simulink model "Controle_UDP_0809_simulador"  (R2014a)
settings: Solver=ode45  StartTime=0.0  StopTime=360  RelTol=1e-3
values from neighbouring files (symbols this model uses):
  Arwx = [-B1/J1 Kt/J1 ... (first row only)    [data_ACS_HIL.m]
  Arwy = [-B2/J2 Kt/J2 ... (first row only)    [data_ACS_HIL.m]
  Arwz = [-B3/J3 Kt/J3 ... (first row only)    [data_ACS_HIL.m]
  Brwx = [0 ... (first row only)    [data_ACS_HIL.m]
  Brwy = [0 ... (first row only)    [data_ACS_HIL.m]
  Brwz = [0 ... (first row only)    [data_ACS_HIL.m]
  Crwx = [1 0 ... (first row only)    [data_ACS_HIL.m]
  Crwy = [1 0 ... (first row only)    [data_ACS_HIL.m]
  Crwz = [1 0 ... (first row only)    [data_ACS_HIL.m]
  Drwx = zeros(3,1)    [data_ACS_HIL.m]
  Drwy = zeros(3,1)    [data_ACS_HIL.m]
  Drwz = zeros(3,1)    [data_ACS_HIL.m]
  I1 = 0.000624567    [data_ACS_HIL.m]
  I2 = 0.000624567    [data_ACS_HIL.m]
  I3 = 0.000624567    [data_ACS_HIL.m]
  in1 = [ 10 10 25 30 0 ] * pi / 180    [data_ACS_HIL.m]
  in2 = [ 0 10 10 30 0 ] * pi / 180    [data_ACS_HIL.m]
  in3 = [ 45 -30 30 30 0 ] * pi / 180    [data_ACS_HIL.m]
  Ixx = I( 1, 1 )    [data_ACS_HIL.m]
  Iyy = I( 2, 2 )    [data_ACS_HIL.m]
  Izz = I( 3, 3 )    [data_ACS_HIL.m]
  J1 = I1 + 3e-06    (= 0.000627567)    [data_ACS_HIL.m]
  J2 = I2 + 3e-06    (= 0.000627567)    [data_ACS_HIL.m]
  J3 = I3 + 3e-06    (= 0.000627567)    [data_ACS_HIL.m]
  Ki_x = 1    [data_ACS_HIL.m]
  Ki_y = Ki_x    (= 1)    [data_ACS_HIL.m]
  Ki_z = Ki_x    (= 1)    [data_ACS_HIL.m]
  Kp_x = 0.2    [data_ACS_HIL.m]
  Kp_y = Kp_x    (= 0.2)    [data_ACS_HIL.m]
  Kp_z = Kp_x    (= 0.2)    [data_ACS_HIL.m]
  Kpx = vp * (wn^2) * Ixx    [data_ACS_HIL.m]
  Kpy = vp * (wn^2) * Iyy    [data_ACS_HIL.m]
  Kpz = vp * (wn^2) * Izz    [data_ACS_HIL.m]
  Krx = vr * 2 * Ixx * wn * qsi    [data_ACS_HIL.m]
  Kry = vr * 2 * Iyy * wn * qsi    [data_ACS_HIL.m]
  Krz = vr * 2 * Izz * wn * qsi    [data_ACS_HIL.m]
  mW0 = 0000 / ( 60 / ( 2*pi ) )    (= 0)    [data_ACS_HIL.m]
  Wx0 = [mW0 0]    [data_ACS_HIL.m]
  Wy0 = [mW0 0]    [data_ACS_HIL.m]
  Wz0 = [mW0 0]    [data_ACS_HIL.m]
libraries: aerolibconvert2 x6, simulink x6, etargetslib x4, instrumentlib x4, aerolibutil x4, xpcutilitieslib x2, slrtlib x2, rtwinlib x1, aerolibtransform2 x1, vrlib x1
(part 2 of 2)

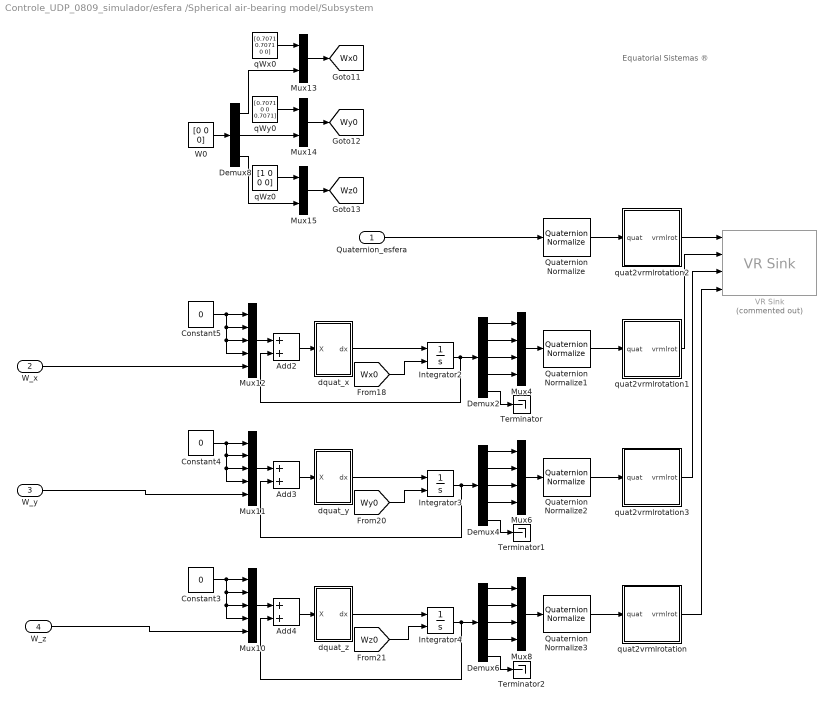
== system Controle_UDP_0809_simulador/esfera /Spherical air-bearing model/Subsystem ==
  note: Equatorial Sistemas ®
  Quaternion_esfera : Inport
  W_x : Inport  Port=2
  W_y : Inport  Port=3
  W_z : Inport  Port=4
  Add2 : Sum
  Add3 : Sum
  Add4 : Sum
  Constant3 : Constant  Value=0
  Constant4 : Constant  Value=0
  Constant5 : Constant  Value=0
  Demux2 : Demux  Outputs=5
  Demux4 : Demux  Outputs=5
  Demux6 : Demux  Outputs=5
  Demux8 : Demux  Outputs=3
  Integrator2 : Integrator  InitialConditionSource=external  InitialCondition=Wx0
  Integrator3 : Integrator  InitialConditionSource=external  InitialCondition=Wy0
  Integrator4 : Integrator  InitialConditionSource=external  InitialCondition=Wz0
  Mux10 : Mux  Inputs=5
  Mux11 : Mux  Inputs=5
  Mux12 : Mux  Inputs=5
  Mux13 : Mux  Inputs=2
  Mux14 : Mux  Inputs=2
  Mux15 : Mux  Inputs=2
  Mux4 : Mux
  Mux6 : Mux
  Mux8 : Mux
  Quaternion Normalize{,1..3} (4 alike) : aerolibutil/Quaternion Normalize
  Terminator : Terminator
  Terminator1 : Terminator
  Terminator2 : Terminator
  VR Sink : vrlib/VR Sink  Commented=on  InstantiateOnLoad=on  SampleTime=0.1  ViewEnable=on  RemoteChange=off  RemoteView=off  FieldsWritten=Corpo.rotation.4.1.1.double#Roda_x.rotation.4.1.1.double#Roda_y.rotation.4.1.1.double#Roda_z.rotation.4.1.1.double  WorldFileName=wrlfiles\esfera_v2.wrl  WorldDescription=VRML MATLAB Membrane  AutoView=on  VideoDimensions=[]  AllowVariableSize=off
  W0 : Constant  Value=[0 0 0]
  dquat_x : Subsystem
  dquat_y : Subsystem
  dquat_z : Subsystem
  qWx0 : Constant  Value=[0.7071 0.7071 0 0]
  qWy0 : Constant  Value=[0.7071 0 0 0.7071]
  qWz0 : Constant  Value=[1 0 0 0]
  quat2vrmlrotation : Subsystem
  quat2vrmlrotation1 : Subsystem
  quat2vrmlrotation2 : Subsystem
  quat2vrmlrotation3 : Subsystem
  tag scope: Wx0=global, Wy0=global, Wz0=global
  wires:
  Integrator2/1 -> Demux2/1, Add2/2
  Mux4/1 -> Quaternion Normalize1/1
  Add2/1 -> dquat_x/1(X)
  Demux2/1 -> Mux4/1
  Demux2/2 -> Mux4/2
  Demux2/3 -> Mux4/3
  Demux2/4 -> Mux4/4
  Integrator3/1 -> Demux4/1, Add3/2
  Mux6/1 -> Quaternion Normalize2/1
  Demux4/1 -> Mux6/1
  Demux4/2 -> Mux6/2
  Demux4/3 -> Mux6/3
  Demux4/4 -> Mux6/4
  Integrator4/1 -> Add4/2, Demux6/1
  Mux8/1 -> Quaternion Normalize3/1
  Quaternion Normalize3/1 -> quat2vrmlrotation/1(quat)
  Demux6/1 -> Mux8/1
  Demux6/2 -> Mux8/2
  Demux6/3 -> Mux8/3
  Demux6/4 -> Mux8/4
  Mux10/1 -> Add4/1
  Mux11/1 -> Add3/1
  Constant5/1 -> Mux12/1, Mux12/2, Mux12/3, Mux12/4
  Mux12/1 -> Add2/1
  Constant4/1 -> Mux11/1, Mux11/2, Mux11/3, Mux11/4
  Constant3/1 -> Mux10/1, Mux10/2, Mux10/3, Mux10/4
  [Wx0] -> Integrator2/2
  [Wy0] -> Integrator3/2
  [Wz0] -> Integrator4/2
  W0/1 -> Demux8/1
  qWx0/1 -> Mux13/1
  Demux8/1 -> Mux13/2
  Mux13/1 -> [Wx0]
  qWy0/1 -> Mux14/1
  Demux8/2 -> Mux14/2
  Mux14/1 -> [Wy0]
  qWz0/1 -> Mux15/1
  Demux8/3 -> Mux15/2
  Mux15/1 -> [Wz0]
  dquat_x/1(dx) -> Integrator2/1
  Add3/1 -> dquat_y/1(X)
  dquat_y/1(dx) -> Integrator3/1
  Add4/1 -> dquat_z/1(X)
  dquat_z/1(dx) -> Integrator4/1
  Demux2/5 -> Terminator/1
  Demux4/5 -> Terminator1/1
  Demux6/5 -> Terminator2/1
  Quaternion Normalize/1 -> quat2vrmlrotation2/1(quat)
  Quaternion Normalize1/1 -> quat2vrmlrotation1/1(quat)
  Quaternion Normalize2/1 -> quat2vrmlrotation3/1(quat)
  quat2vrmlrotation2/1(vrmlrot) -> VR Sink/1
  quat2vrmlrotation1/1(vrmlrot) -> VR Sink/2
  quat2vrmlrotation3/1(vrmlrot) -> VR Sink/3
  quat2vrmlrotation/1(vrmlrot) -> VR Sink/4
  W_y/1 -> Mux11/5
  W_z/1 -> Mux10/5
  W_x/1 -> Mux12/5
  Quaternion_esfera/1 -> Quaternion Normalize/1

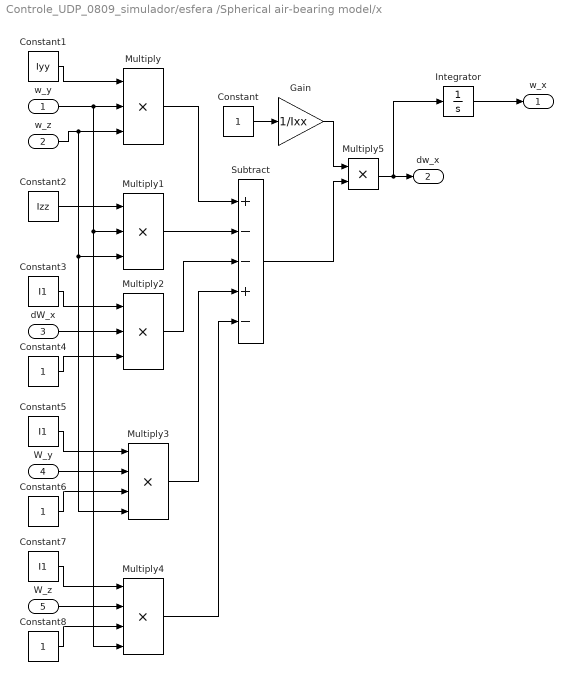
== system Controle_UDP_0809_simulador/esfera /Spherical air-bearing model/x ==
  w_y : Inport
  w_z : Inport  Port=2
  dW_x : Inport  Port=3
  W_y : Inport  Port=4
  W_z : Inport  Port=5
  Constant{,4,6,8} (4 alike) : Constant
  Constant1 : Constant  Value=Iyy
  Constant2 : Constant  Value=Izz
  Constant3 : Constant  Value=I1
  Constant5 : Constant  Value=I1
  Constant7 : Constant  Value=I1
  Gain : Gain  Gain=1/Ixx
  Integrator : Integrator
  Multiply : Product  Inputs=***
  Multiply1 : Product  Inputs=***
  Multiply2 : Product  Inputs=***
  Multiply3 : Product  Inputs=****
  Multiply4 : Product  Inputs=****
  Multiply5 : Product  Inputs=**
  Subtract : Sum  Inputs=+--+-
  w_x : Outport
  dw_x : Outport  Port=2
  wires:
  Constant/1 -> Gain/1
  Gain/1 -> Multiply5/1
  Constant1/1 -> Multiply/1
  Multiply/1 -> Subtract/1
  Constant2/1 -> Multiply1/1
  Multiply1/1 -> Subtract/2
  Constant3/1 -> Multiply2/1
  Constant4/1 -> Multiply2/3
  Multiply2/1 -> Subtract/3
  Constant5/1 -> Multiply3/1
  Constant6/1 -> Multiply3/3
  Constant7/1 -> Multiply4/1
  Constant8/1 -> Multiply4/3
  Multiply3/1 -> Subtract/4
  Multiply4/1 -> Subtract/5
  Subtract/1 -> Multiply5/2
  w_y/1 -> Multiply/2, Multiply1/2, Multiply4/4
  w_z/1 -> Multiply/3, Multiply1/3, Multiply3/4
  dW_x/1 -> Multiply2/2
  W_y/1 -> Multiply3/2
  W_z/1 -> Multiply4/2
  Multiply5/1 -> Integrator/1, dw_x/1
  Integrator/1 -> w_x/1

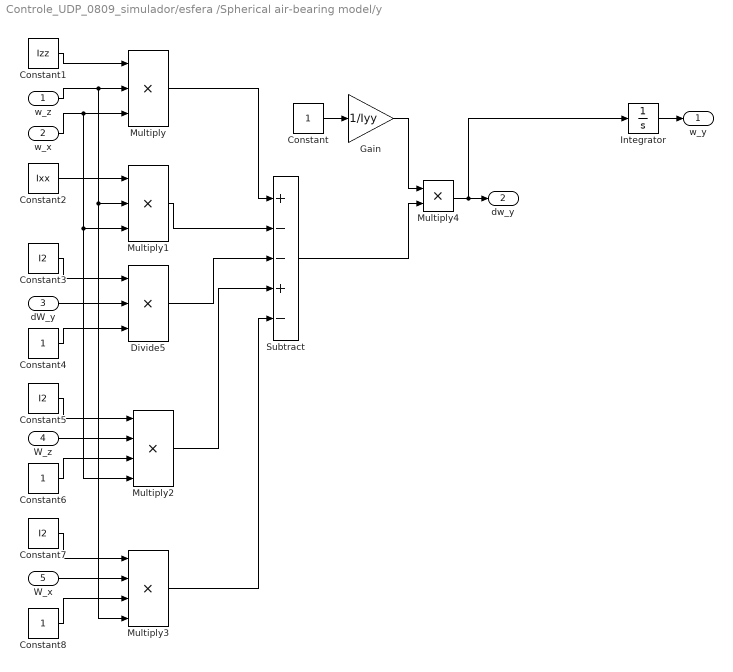
== system Controle_UDP_0809_simulador/esfera /Spherical air-bearing model/y ==
  w_z : Inport
  w_x : Inport  Port=2
  dW_y : Inport  Port=3
  W_z : Inport  Port=4
  W_x : Inport  Port=5
  Constant{,4,6,8} (4 alike) : Constant
  Constant1 : Constant  Value=Izz
  Constant2 : Constant  Value=Ixx
  Constant3 : Constant  Value=I2
  Constant5 : Constant  Value=I2
  Constant7 : Constant  Value=I2
  Divide5 : Product  Inputs=***
  Gain : Gain  Gain=1/Iyy
  Integrator : Integrator
  Multiply : Product  Inputs=***
  Multiply1 : Product  Inputs=***
  Multiply2 : Product  Inputs=****
  Multiply3 : Product  Inputs=****
  Multiply4 : Product  Inputs=**
  Subtract : Sum  Inputs=+--+-
  w_y : Outport
  dw_y : Outport  Port=2
  wires:
  W_x/1 -> Multiply3/2
  W_z/1 -> Multiply2/2
  dW_y/1 -> Divide5/2
  w_x/1 -> Multiply2/4, Multiply1/3, Multiply/3
  w_z/1 -> Multiply3/4, Multiply1/2, Multiply/2
  Subtract/1 -> Multiply4/2
  Multiply3/1 -> Subtract/5
  Multiply2/1 -> Subtract/4
  Constant8/1 -> Multiply3/3
  Constant7/1 -> Multiply3/1
  Constant6/1 -> Multiply2/3
  Constant5/1 -> Multiply2/1
  Divide5/1 -> Subtract/3
  Constant4/1 -> Divide5/3
  Constant3/1 -> Divide5/1
  Multiply1/1 -> Subtract/2
  Constant2/1 -> Multiply1/1
  Multiply/1 -> Subtract/1
  Constant1/1 -> Multiply/1
  Integrator/1 -> w_y/1
  Gain/1 -> Multiply4/1
  Constant/1 -> Gain/1
  Multiply4/1 -> Integrator/1, dw_y/1

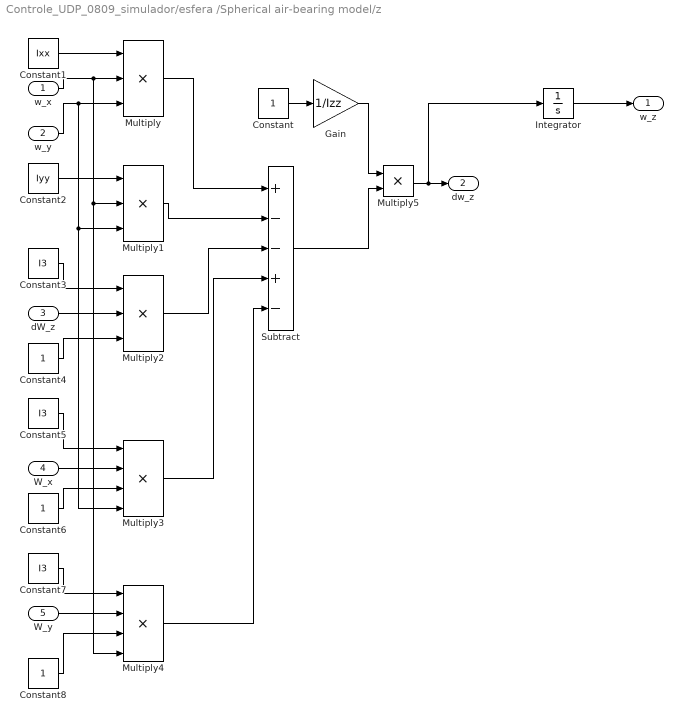
== system Controle_UDP_0809_simulador/esfera /Spherical air-bearing model/z ==
  w_x : Inport
  w_y : Inport  Port=2
  dW_z : Inport  Port=3
  W_x : Inport  Port=4
  W_y : Inport  Port=5
  Constant{,4,6,8} (4 alike) : Constant
  Constant1 : Constant  Value=Ixx
  Constant2 : Constant  Value=Iyy
  Constant3 : Constant  Value=I3
  Constant5 : Constant  Value=I3
  Constant7 : Constant  Value=I3
  Gain : Gain  Gain=1/Izz
  Integrator : Integrator
  Multiply : Product  Inputs=***
  Multiply1 : Product  Inputs=***
  Multiply2 : Product  Inputs=***
  Multiply3 : Product  Inputs=****
  Multiply4 : Product  Inputs=****
  Multiply5 : Product  Inputs=**
  Subtract : Sum  Inputs=+--+-
  w_z : Outport
  dw_z : Outport  Port=2
  wires:
  Constant/1 -> Gain/1
  Gain/1 -> Multiply5/1
  Integrator/1 -> w_z/1
  Constant1/1 -> Multiply/1
  Multiply/1 -> Subtract/1
  Constant2/1 -> Multiply1/1
  Multiply1/1 -> Subtract/2
  Constant3/1 -> Multiply2/1
  Constant4/1 -> Multiply2/3
  Multiply2/1 -> Subtract/3
  Constant5/1 -> Multiply3/1
  Constant6/1 -> Multiply3/3
  Constant7/1 -> Multiply4/1
  Constant8/1 -> Multiply4/3
  Multiply3/1 -> Subtract/4
  Multiply4/1 -> Subtract/5
  Subtract/1 -> Multiply5/2
  w_x/1 -> Multiply/2, Multiply1/2, Multiply4/4
  w_y/1 -> Multiply/3, Multiply1/3, Multiply3/4
  dW_z/1 -> Multiply2/2
  W_x/1 -> Multiply3/2
  W_y/1 -> Multiply4/2
  Multiply5/1 -> Integrator/1, dw_z/1

== system Controle_UDP_0809_simulador/controle /Logica de controle/Logica de Controle/subtrator de angulos ==
  + : Inport
  - : Inport  Port=2
  Constant2 : Constant  Value=2*pi
  Gain : Gain  Gain=-1
  Sum : Sum  Inputs=|+-
  Sum1 : Sum  Inputs=|+-
  Sum2 : Sum  Inputs=|++
  Switch : Switch  Criteria=u2 > Threshold  Threshold=180*pi/180
  Switch1 : Switch  Criteria=u2 > Threshold  Threshold=180*pi/180
  Out1 : Outport
  wires:
  Sum2/1 -> Switch1/1
  Gain/1 -> Switch1/2
  Sum/1 -> Switch/3, Switch/2, Sum1/1
  Sum1/1 -> Switch/1
  Switch/1 -> Switch1/3, Gain/1, Sum2/1
  Constant2/1 -> Sum1/2, Sum2/2
  Switch1/1 -> Out1/1
  -/1 -> Sum/2
  +/1 -> Sum/1

== system Controle_UDP_0809_simulador/esfera /Spherical air-bearing model/Subsystem/dquat_x ==
  X : Inport
  Constant : Constant  Value=0
  Demux : Demux  Outputs=5
  Gain : Gain  Gain=1/2
  Gain1 : Gain  Gain=-1
  Gain2 : Gain  Gain=-1
  Mux : Mux  Inputs=5
  Product{,1..3} (4 alike) : Product
  dx : Outport
  wires:
  X/1 -> Gain/1
  Gain1/1 -> Product/1
  Product1/1 -> Mux/2
  Product2/1 -> Mux/3
  Product3/1 -> Mux/4
  Gain/1 -> Demux/1
  Product/1 -> Mux/1
  Demux/5 -> Product/2, Product1/2, Product2/2, Product3/2
  Mux/1 -> dx/1
  Constant/1 -> Mux/5
  Demux/3 -> Gain1/1
  Gain2/1 -> Product1/1
  Demux/4 -> Gain2/1
  Demux/1 -> Product2/1
  Demux/2 -> Product3/1

== system Controle_UDP_0809_simulador/esfera /Spherical air-bearing model/Subsystem/dquat_y ==
  X : Inport
  Constant : Constant  Value=0
  Demux : Demux  Outputs=5
  Gain : Gain  Gain=1/2
  Gain1 : Gain  Gain=-1
  Gain2 : Gain  Gain=-1
  Mux : Mux  Inputs=5
  Product{,1..3} (4 alike) : Product
  dx : Outport
  wires:
  X/1 -> Gain/1
  Gain1/1 -> Product/1
  Product1/1 -> Mux/2
  Product2/1 -> Mux/3
  Product3/1 -> Mux/4
  Gain/1 -> Demux/1
  Product/1 -> Mux/1
  Demux/5 -> Product/2, Product1/2, Product2/2, Product3/2
  Mux/1 -> dx/1
  Constant/1 -> Mux/5
  Demux/3 -> Gain1/1
  Gain2/1 -> Product1/1
  Demux/4 -> Gain2/1
  Demux/1 -> Product2/1
  Demux/2 -> Product3/1

== system Controle_UDP_0809_simulador/esfera /Spherical air-bearing model/Subsystem/dquat_z ==
  X : Inport
  Constant : Constant  Value=0
  Demux : Demux  Outputs=5
  Gain : Gain  Gain=1/2
  Gain1 : Gain  Gain=-1
  Gain2 : Gain  Gain=-1
  Mux : Mux  Inputs=5
  Product{,1..3} (4 alike) : Product
  dx : Outport
  wires:
  X/1 -> Gain/1
  Gain1/1 -> Product/1
  Product1/1 -> Mux/2
  Product2/1 -> Mux/3
  Product3/1 -> Mux/4
  Demux/1 -> Product2/1
  Demux/3 -> Gain1/1
  Demux/2 -> Gain2/1
  Gain2/1 -> Product3/1
  Gain/1 -> Demux/1
  Product/1 -> Mux/1
  Demux/5 -> Product/2, Product1/2, Product2/2, Product3/2
  Mux/1 -> dx/1
  Demux/4 -> Product1/1
  Constant/1 -> Mux/5

== system Controle_UDP_0809_simulador/esfera /Spherical air-bearing model/Subsystem/quat2vrmlrotation ==
  quat : Inport
  Fcn1 : Fcn  Expr=u(2)/(sin(2*acos(u(1))/2))
  Fcn2 : Fcn  Expr=u(3)/(sin(2*acos(u(1))/2))
  Fcn3 : Fcn  Expr=2*acos(u(1))
  Fcn4 : Fcn  Expr=u(4)/(sin(2*acos(u(1))/2))
  Mux9 : Mux
  vrmlrot : Outport
  wires:
  Mux9/1 -> vrmlrot/1
  Fcn3/1 -> Mux9/4
  Fcn1/1 -> Mux9/1
  quat/1 -> Fcn3/1, Fcn1/1, Fcn2/1, Fcn4/1
  Fcn2/1 -> Mux9/2
  Fcn4/1 -> Mux9/3

== system Controle_UDP_0809_simulador/esfera /Spherical air-bearing model/Subsystem/quat2vrmlrotation1 ==
  quat : Inport
  Fcn1 : Fcn  Expr=u(2)/(sin(2*acos(u(1))/2))
  Fcn2 : Fcn  Expr=u(3)/(sin(2*acos(u(1))/2))
  Fcn3 : Fcn  Expr=2*acos(u(1))
  Fcn4 : Fcn  Expr=u(4)/(sin(2*acos(u(1))/2))
  Mux9 : Mux
  vrmlrot : Outport
  wires:
  Fcn4/1 -> Mux9/3
  Fcn2/1 -> Mux9/2
  quat/1 -> Fcn4/1, Fcn2/1, Fcn1/1, Fcn3/1
  Fcn1/1 -> Mux9/1
  Fcn3/1 -> Mux9/4
  Mux9/1 -> vrmlrot/1

== system Controle_UDP_0809_simulador/esfera /Spherical air-bearing model/Subsystem/quat2vrmlrotation2 ==
  quat : Inport
  Fcn1 : Fcn  Expr=-u(3)/(sin(2*acos(u(1))/2))
  Fcn2 : Fcn  Expr=-u(2)/(sin(2*acos(u(1))/2))
  Fcn3 : Fcn  Expr=2*acos(u(1))
  Fcn4 : Fcn  Expr=u(4)/(sin(2*acos(u(1))/2))
  Mux9 : Mux
  vrmlrot : Outport
  wires:
  Mux9/1 -> vrmlrot/1
  Fcn3/1 -> Mux9/4
  quat/1 -> Fcn3/1, Fcn1/1, Fcn2/1, Fcn4/1
  Fcn4/1 -> Mux9/3
  Fcn1/1 -> Mux9/1
  Fcn2/1 -> Mux9/2

== system Controle_UDP_0809_simulador/esfera /Spherical air-bearing model/Subsystem/quat2vrmlrotation3 ==
  quat : Inport
  Fcn1 : Fcn  Expr=u(2)/(sin(2*acos(u(1))/2))
  Fcn2 : Fcn  Expr=u(3)/(sin(2*acos(u(1))/2))
  Fcn3 : Fcn  Expr=2*acos(u(1))
  Fcn4 : Fcn  Expr=u(4)/(sin(2*acos(u(1))/2))
  Mux9 : Mux
  vrmlrot : Outport
  wires:
  Mux9/1 -> vrmlrot/1
  Fcn3/1 -> Mux9/4
  Fcn1/1 -> Mux9/1
  quat/1 -> Fcn3/1, Fcn1/1, Fcn2/1, Fcn4/1
  Fcn2/1 -> Mux9/2
  Fcn4/1 -> Mux9/3

== matlab function Controle_UDP_0809_simulador/esfera /Spherical air-bearing model/MATLAB Function ==
  data: x input; dq output
function dq = dquat( x )
K = 0.00001;

w = x( 1:3 );

q = x( 4:7 );

ep = 1 - q(1)^2 + q(2)^2 + q(3)^2 + q(4)^2;

dq = ( 1/2 ) * [    0 -w(1) -w(2) -w(3);
                 w(1)     0  w(3) -w(2);
                 w(2) -w(3)     0  w(1);
                 w(3)  w(2) -w(1)     0;] * q + K * ep * q;
return
